simulink model "Source_Dev"  (R2020a)
settings: Solver=ode1  StartTime=0.0  StopTime=3  FixedStep=Time_Step  RelTol=1e-3
values from neighbouring files (symbols this model uses):
  fb = fn    (= 50)    [init.m]
  L0102_L = L0102_X/wb    (= 0.254647908947)    [init.m]
  L0102_R = L0102_R_u*L0102_Zb    (= 8)    [init.m]
  Time_Step = 50e-6    (= 5e-05)    [init.m]
undefined symbols (not defined in the file or in its folder): GRD00_H, GRD00_R, GRD00_TD, GRD00_TN, GRD00_Ub, Source_Lib, Theta0, ThreePhaseVoltageSource, V0, VSC01_id0
libraries: powerlib x54, Control_Lib x6, simulink x5, powerlib_meascontrol x2
(part 1 of 2)
settings Model: Creator=abruyere  LastModifiedBy=abruyere
settings DebuggingCC: UnconnectedInputMsg=none  UnconnectedOutputMsg=none  UnconnectedLineMsg=none
settings SFSimCC: CustomCodeUndefinedFunction=UseInterfaceOnly

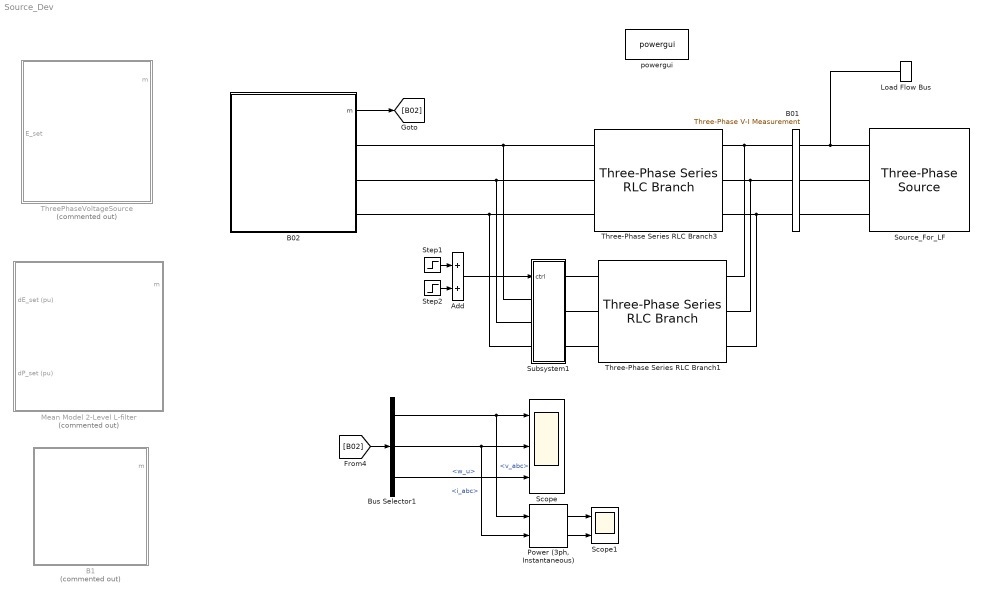
== system Source_Dev ==
  Add : Sum
  B01 : powerlib/Measurements/Three-Phase V-I Measurement  VoltageMeasurement=phase-to-ground  SetLabelV=on  LabelV=B01_v_abc  Vpu=off  VpuLL=off  CurrentMeasurement=yes  SetLabelI=on  LabelI=B01_i_abc  Ipu=off  Pbase=100e6  Vbase=500e3  OutputType=Complex  PhasorSimulation=off  PSBequivalent=0
  B02 : Subsystem  mask(GenericVoltageSource){SourceNature=2 % INERTIAL, fn=50, Sn=10000e3, Un=20000, LFpopup=PQ, P0=350000.4063, Q0=2.0599, U0=10000, V0_pu=1.0045, Theta0_deg=3.9958, H_s=5, R_percent=4, TN=1, TD=2}
      mask prompts: SourceNature "Nature of the source: Choose 1 for infinite source or 2 for inertial source"; fn "Nominal frequency fn [Hz]"; Sn "Nominal apparent power Sn [VA]"; Un "Base nominal voltage Un [V RMS Ph2Ph]"; P0 "Active power P0 [W]"; Q0 "Reactive power Q0 [VAR]"; U0 "Initial voltage U0 [Vrms Ph2Ph]"; V0_pu "Initial pu voltage V0_pu [pu]"; Theta0_deg "Initial angle (°)"; H_s "Inertia H [s]"; R_percent "Droop gain Kp [%]"; TN "Network time constant Lead [s]"; TD "Network time constant Lag [s]"
      mask init:
      | % Update Name of LF bus for internal purpose
      | NameStr = [get_param(gcb,'Name')];% '_LF'];
      | set_param([gcb '/Load Flow Bus'],'ID',NameStr);  
      | 
      | % Base specification
      | fb = fn;                % [Hz] base frequency
      | Sb = Sn;                % [VA] base power
      | Ub = Un;                % [V] base ph2ph voltage
      | Vb = Un/sqrt(3);        % [V] base ph2N voltage
      | Ib = Sb/(3*Vb);         % [A] base current
      | Zb = Vb*Ib;             % [Ohm] base impedance
      | 
      | % Set the frequency droop gain
      | R = R_percent / 100;
      | 
      | % Update mask display:
      | % mo = get_param(gcb,'MaskObject');
      settings: OpenFcn=|
      | set_param(gcb,'MaskType', 'GenericVoltageSource')
      | open_system(gcbh, 'Mask');
      mask TypeOptions SourceNature: 1 % INIFINTE | 2 % INERTIAL
      mask TypeOptions LFpopup: Swing | PQ | PV
      mask Callback LFpopup:
      | % Get the mask parameter values. This is a cell
      | %   array of character vectors.
      | maskStr = get_param(gcb,'LFpopup');
      | p=Simulink.Mask.get(gcb);
      | 
      | % The pop-up menu is the first mask parameter.
      | %   Check the value selected in the pop-up
      | if strcmp(maskStr,'Swing'),
      | 
      |     % Set the visibility of both parameters on when
      |     %   User-defined is selected in the pop-up.
      |     p.getParameter('P0').Visible='off';
      |     p.getParameter('Q0').Visible='off';
      |     p.getParameter('U0').Visible='on';
      |     p.getParameter('Theta0_deg').Visible='on';
      |     set_param([gcb '/Source_For_LF'],'BusType','swing');
      | 
      | elseif strcmp(maskStr,'PQ'),
      | 
      |     % Set the visibility of both parameters on when
      |     %   User-defined is selected in the pop-up.
      |     p.getParameter('P0').Visible='on';
      |     p.getParameter('Q0').Visible='on';
      |     p.getParameter('U0').Visible='off';
      |     p.getParameter('Theta0_deg').Visible='on';
      |     set_param([gcb '/Source_For_LF'],'BusType','PQ');
      | 
      |     % Turn off the visibility of the Value field
      |     %   when User-defined is not selected.
      | else
      | 
      |     % Set the visibility of both parameters on when
      |     %   User-defined is selected in the pop-up.
      |     p.getParameter('P0').Visible='on';
      |     p.getParameter('Q0').Visible='off';
      |     p.getParameter('U0').Visible='on';
      |     p.getParameter('Theta0_deg').Visible='on';
      |     set_param([gcb '/Source_For_LF'],'BusType','PV');
      | 
      | end
      mask DialogControl Container2 Prompt: Nominal specification (for base definition)
      mask DialogControl Container3 Prompt: Loadflow specification
      mask DialogControl Container4_copy Prompt: Inertial source configuration
  B1 : Subsystem  Commented=on  mask(GenericVoltageSource){SourceNature=2 % INERTIAL, fn=50, Sn=1000e3, Un=20e3, P0=199999.317, Q0=4.3832, H_s=5, R_percent=5, V0_pu=0.99767, Theta0_deg=4.0629}
      mask prompts: SourceNature "Nature of the source: Choose 1 for infinite source or 2 for inertial source"; fn "Nominal frequency fn [Hz]"; Sn "Nominal apparent power Sn [VA]"; Un "Base nominal voltage Un [V RMS Ph2Ph]"; P0 "Active power P0 [W]"; Q0 "Reactive power Q0 [VAR]"; H_s "Inertia H [s]"; R_percent "Droop gain Kp [%]"; V0_pu "V0 [pu]"; Theta0_deg "Theta0 [°]"
      mask init:
      | % Update Name of LF bus for internal purpose
      | NameStr = [get_param(gcb,'Name')];% '_LF'];
      | set_param([gcb '/Load Flow Bus'],'ID',NameStr);  
      | 
      | % Base specification
      | fb = fn;                % [Hz] base frequency
      | Sb = Sn;                % [VA] base power
      | Ub = Un;                % [V] base ph2ph voltage
      | Vb = Un/sqrt(3);        % [V] base ph2N voltage
      | Ib = Sb/(3*Vb);         % [A] base current
      | Zb = Vb*Ib;             % [Ohm] base impedance
      | 
      | % Set the frequency droop gain
      | R = R_percent / 100;
      | 
      | % Update mask display:
      | mo = get_param(gcb,'MaskObject');
      | % mo.getDialogControl('LF_V0_str').Prompt = ['V0 = ', num2str(V0),' pu, Angle = ', num2str(V0),'°'];
      settings: OpenFcn=|
      | set_param(gcb,'MaskType', 'GenericVoltageSource')
      | open_system(gcbh, 'Mask');
      mask TypeOptions SourceNature: 1 % INIFINTE | 2 % INERTIAL
      mask DialogControl Container2 Prompt: Nominal specification (for base definition)
      mask DialogControl Container3 Prompt: Setpoint specification (for loadflow)
      mask DialogControl Container4_copy Prompt: Inertial source configuration
      mask DialogControl Container4 Prompt: Info
  Bus Selector1 : BusSelector  OutputSignals=v_abc,i_abc,w_u
  Load Flow Bus : powerlib/Measurements/Load Flow Bus  LConnTagsString=a  Phases=single  Connectors=on one side  ID=B01  Vbase=20e3  Vref=1  Vangle=0  VLF=1  VLFb=1  VLFc=1  angleLF=0  angleLFb=0  angleLFc=0
  Mean Model 2-Level L-filter : Subsystem  Commented=on  AncestorBlock=GFo_Lib/Mean Model 2-Level L-filter  mask(VSC){Parameter33=0, fn=50, Sn=1000e6, Pn=1000e6, Udcn=640e3, Un1=320e3, Un2=400e3, Rt_pu=0.005, Lt_pu=0.15, Lm_pu=500, Rm_pu=500, Tr_PLL=10e-3, Val_Freq_Support=on, R_percent=4, Rv=0.009, W_TVR=60, I_thresh_pu=1, DX_DR=5, Kp_Rvi_pu=0.676, gainpopup=3, wc1=31.4159, mp1=0.0043, wc2=33.3, mp2=0.0033, wc3=2.5, mp3=0.04, T1=0.1210, T2=0.022, LFpopup=PQ, P0=0.5, Q0=0.1, V0=1.0246, Theta0=118.5692}
      mask prompts: Parameter33 "%<MaskType>"; fn "Nominal Frequency (Hz)"; Sn "Nominal Apparent Power (VA)"; Pn "Nominal Power (W)"; Udcn "Nominal DC Voltage (V)"; Un1 "VSC side Nominal Ph-Ph Voltage (V)"; Un2 "Grid side Nominal Ph-Ph Voltage (V)"; Rt_pu "R (pu)"; Lt_pu "L (pu)"; Lm_pu "Rm (pu)"; Rm_pu "Lm (pu)"; Tr_PLL "Time response (s)"; Val_Freq_Support "Frequency Support"; R_percent "Droop Gain (%)"; Rv "Damping Resistance (Rv)"; W_TVR "Dr filter"; I_thresh_pu "Current Threshold (pu)"; Kp_Rvi_pu "Kp_Rvi"; gainpopup "Strategy"; wc1 "wc"; mp1 "mp"; wc2 "wc"; mp2 "mp"; wc3 "wc"; mp3 "mp"; P0 "Initial Active Power (pu)"; Q0 "Initial Reactive Power (pu)"; V0 "Initial Voltage (pu)"; Theta0 "Initial Angle (°)"
      mask init:
      | % Update Name of LF bus for internal purpose
      |     NameStr = [get_param(gcb,'Name')];% '_LF'];
      |     set_param([gcb '/Load Flow Bus'],'ID',NameStr);    
      |     
      | % Base values
      |     fb = fn;
      |     Pb = Pn;
      |     cos_phi_n = Pn/Sn;
      |     Sb = Pb/cos_phi_n;
      |     Vn1 = Un1/sqrt(3);
      |     Vb1 = Vn1;
      |     Vn2 = Un2/sqrt(3);
      |     Vb2 = Vn2;
      |     Ib1 = Sb / 3*Vb1;
      |     Ib2 = Sb / (3*Vb2);
      |     wb = 2*pi*fb;
      |   
      | % PLL derivation of the parameters
      |     wn_PLL=5/Tr_PLL;
      |     zeta_PLL = 1;
      |     Kp_PLL_pu = 2*zeta_PLL*wn_PLL/wb;
      |     Ki_PLL_pu = wn_PLL^2/wb;
      |     
      | % Set the chosen strategy
      |     Chosen_Strategy = gainpopup;
      |     
      | % Set the frequency droop gain
      |     R = R_percent / 100;
      | 
      | % Compute Initial Voltage of VSC 
      | %   from steady-state output transformer model and Loadflow result
      |     
      |     %Initialize correctly the LoadFlow bus parameters connected to PCC
      |     VLF = V0;
      |     ThetaLF = Theta0;
      |     if (LFpopup == 'PQ')
      |         VLF = 1;
      |         ThetaLF = 0;
      |     elseif (LFpopup == 'PV')
      |         VLF = V0;
      |         ThetaLF = 0;        
      |     end
      |     set_param([gcb '/Load Flow Bus'],'Vref',num2str(VLF),'Vangle',num2str(ThetaLF));
      |     
      |     R1_pu = Rt_pu/2;
      |     L1_pu = Lt_pu/2;
      |     R2_pu = Rt_pu/2;
      |     L2_pu = Lt_pu/2;
      |     X1_pu = L1_pu;
      |     X2_pu = L2_pu;
      |     Xm_pu = Lm_pu;
      |     
      |     Zm_pu = 1/(1/Rm_pu+1/(1i*Xm_pu));
      | 
      |     S0=P0+1i*Q0;
      |     I2 = conj(S0)/(V0);
      | 
      |     Vm = (R2_pu+1i*X2_pu)*I2 + V0;
      |     Im = Vm/Zm_pu;
      | 
      |     I1 = I2 + Im;
      |     V1 = (R1_pu+1i*X1_pu) * I1 + Vm;
      | 
      |     Vvsc0 = abs(V1);
      |     Theta_vsc0 = angle(V1) * 180/pi+Theta0;
      |     
      |     Va0 = Vvsc0*sqrt(2)*Vb1*sin(Theta_vsc0*pi/180);
      |     Vb0 = Vvsc0*sqrt(2)*Vb1*sin(Theta_vsc0*pi/180-2*pi/3);
      |     Vc0 = Vvsc0*sqrt(2)*Vb1*sin(Theta_vsc0*pi/180+2*pi/3);
      |     
      | % Generate string to display LF results on Mask
      |     %str_tmp = fprintf("Vvsc0 = %d, Theta_vsc0 = %d°",Vvsc0,Theta_vsc0);
      |     mo = get_param(gcb,'MaskObject');
      |     mo.getDialogControl('LF_vsc_str').Prompt = ['V0 = ', num2str(Vvsc0),' pu, Angle = ', num2str(Theta_vsc0),'°'];
      |     mo.getDialogControl('LF_pcc_str').Prompt = ['V0 = ', num2str(V0),' pu, Angle = ', num2str(Theta0),'°'];
      |     mo.getDialogControl('LF_pcc_Power_str').Prompt = ['P0 = ', num2str(P0),' pu, Q0 = ', num2str(Q0),' pu'];
      |     %set_param([gcb],'LF_str',str_tmp);
      settings: OpenFcn=|
      | NameStr = get_param(gcb,'Name');
      | open_system(gcbh, 'Mask');
      | 
      | h2AllOpenDlgs = DAStudio.ToolRoot.getOpenDialogs;
      | 
      | for i=1:length(h2AllOpenDlgs)
      |     try
      |          %disp(h2AllOpenDlgs(i).getSource.getBlock.Name);
      |         Dialog_block_name = h2AllOpenDlgs(i).getSource.getBlock.Name;
      |          %strcmp(Dialog_block_name, NameStr),
      |         if (strcmp(h2AllOpenDlgs(i).getSource.getBlock.Name, NameStr))
      |             iPos = h2AllOpenDlgs(i).position;
      |             h2AllOpenDlgs(i).position = [iPos(1)   iPos(2)   iPos(3)*1.4   iPos(4)];
      |         end
      |     end
      | end
      mask TypeOptions gainpopup: 1 | 2 | 3
      mask Callback gainpopup:
      | % Get the mask parameter values. This is a cell
      | %   array of character vectors.
      | maskStr = get_param(gcb,'gainpopup');
      | p=Simulink.Mask.get(gcb);
      | 
      | % The pop-up menu is the first mask parameter.
      | %   Check the value selected in the pop-up
      | if strcmp(maskStr,'1'),
      | 
      |     % Set the visibility of both parameters on when
      |     %   User-defined is selected in the pop-up.
      |     p.getDialogControl('Param_Strat_1').Visible='on';
      |     p.getDialogControl('Param_Strat_2').Visible='off';
      |     p.getDialogControl('Param_Strat_3').Visible='off';
      | 
      | elseif strcmp(maskStr,'2'),
      | 
      |     % Set the visibility of both parameters on when
      |     %   User-defined is selected in the pop-up.
      |     p.getDialogControl('Param_Strat_1').Visible='off';
      |     p.getDialogControl('Param_Strat_2').Visible='on';
      |     p.getDialogControl('Param_Strat_3').Visible='off';
      | 
      |     % Turn off the visibility of the Value field
      |     %   when User-defined is not selected.
      | else
      | 
      |     % Set the visibility of both parameters on when
      |     %   User-defined is selected in the pop-up.
      |     p.getDialogControl('Param_Strat_1').Visible='off';
      |     p.getDialogControl('Param_Strat_2').Visible='off';
      |     p.getDialogControl('Param_Strat_3').Visible='on';
      | 
      | end
      mask TypeOptions LFpopup: Swing | PQ | PV
      mask Callback LFpopup:
      | % Get the mask parameter values. This is a cell
      | %   array of character vectors.
      | maskStr = get_param(gcb,'LFpopup');
      | p=Simulink.Mask.get(gcb);
      | 
      | % The pop-up menu is the first mask parameter.
      | %   Check the value selected in the pop-up
      | if strcmp(maskStr,'Swing'),
      | 
      |     % Set the visibility of both parameters on when
      |     %   User-defined is selected in the pop-up.
      |     p.getParameter('P0').Visible='off';
      |     p.getParameter('Q0').Visible='off';
      |     p.getParameter('V0').Visible='on';
      |     p.getParameter('Theta0').Visible='on';
      |     set_param([gcb '/Source_For_LF'],'BusType','swing');
      | 
      | elseif strcmp(maskStr,'PQ'),
      | 
      |     % Set the visibility of both parameters on when
      |     %   User-defined is selected in the pop-up.
      |     p.getParameter('P0').Visible='on';
      |     p.getParameter('Q0').Visible='on';
      |     p.getParameter('V0').Visible='off';
      |     p.getParameter('Theta0').Visible='off';
      |     set_param([gcb '/Source_For_LF'],'BusType','PQ');
      | 
      |     % Turn off the visibility of the Value field
      |     %   when User-defined is not selected.
      | else
      | 
      |     % Set the visibility of both parameters on when
      |     %   User-defined is selected in the pop-up.
      |     p.getParameter('P0').Visible='on';
      |     p.getParameter('Q0').Visible='off';
      |     p.getParameter('V0').Visible='on';
      |     p.getParameter('Theta0').Visible='off';
      |     set_param([gcb '/Source_For_LF'],'BusType','PV');
      | 
      | end
      mask DialogControl Control8 Prompt: (Add text here and link in callback)
      mask DialogControl Nominal_Param Prompt: Nominal Value
      mask DialogControl Container20 Prompt: Output Transformer
      mask DialogControl Control_Param Prompt: Control Parameter
      mask DialogControl Container13 Prompt: PLL
      mask DialogControl Container14 Prompt: Frequency Support
      mask DialogControl Container15 Prompt: Transient Virtual Resistor
      mask DialogControl Container28 Prompt: Virtual Impedance
      mask DialogControl Container18 Prompt: Control Strategy
      mask DialogControl Title_Strat_1 Prompt: Strategy 1
      mask DialogControl Title_Strat_2 Prompt: Strategy 2
      mask DialogControl Title_Strat_3 Prompt: Strategy 3
      mask DialogControl LF_Param Prompt: Loadflow
      mask DialogControl Control4 Prompt: Initial Operating Point
      mask DialogControl Container24 Prompt: VSC side
      mask DialogControl LF_vsc_str Prompt: V0 = 1.0444 pu, Angle = 122.57°
      mask DialogControl Container25 Prompt: PCC
      mask DialogControl LF_pcc_str Prompt: V0 = 1.0246 pu, Angle = 118.5692°
      mask DialogControl LF_pcc_Power_str Prompt: P0 = 0.5 pu, Q0 = 0.1 pu
      mask DialogControl UpdateLoadflow Prompt: Update Loadflow
      mask DialogControl UpdateLoadflow Callback: LoadFlow_VSC
      mask Display:
      | disp('L-Filter');
      | port_label('input',1,'dE_set (pu)');
      | port_label('input',2,'dP_set (pu)');
      | port_label('output',1,'m');
      | port_label('rconn',1,'A');
      | port_label('rconn',2,'B');
      | port_label('rconn',3,'C');
  "Power (3ph, Instantaneous)" : powerlib_meascontrol/Measurements/Power (3ph, Instantaneous)
  Scope : Scope  NumInputPorts=3
  Scope1 : Scope  NumInputPorts=2
  Source_For_LF : powerlib/Electrical Sources/Three-Phase Source  InternalConnection=Yg  VoltagePhases=off  Voltage=(20000)*1  PhaseAngle=0  Voltage_phases=[25e3 25e3 25e3]/sqrt(3)  PhaseAngles_phases=[0 -120 +120]  Frequency=50  NonIdealSource=off  SpecifyImpedance=off  Resistance=0  Inductance=0  ShortCircuitLevel=100e6  BaseVoltage=GRD00_Un  XRratio=7  BusType=swing  Pref=350e3  Qref=0  Prefabc=[10e3, 10e3, 10e3]  Qrefabc=[0, 0, 0]  Qmin=-inf  Qmax=inf
  Step1 : Step  Time=0.5  Before=1  After=0  SampleTime=0
  Step2 : Step  Time=2  SampleTime=0
  Subsystem1 : Subsystem
  Three-Phase Series RLC Branch1 : powerlib/Elements/Three-Phase Series RLC Branch  LConnTagsString=A|B|C  RConnTagsString=A|B|C  BranchType=RL  Resistance=L0102_R*2  Inductance=L0102_L*2  Capacitance=1e-6  Measurements=None
  Three-Phase Series RLC Branch3 : powerlib/Elements/Three-Phase Series RLC Branch  LConnTagsString=A|B|C  RConnTagsString=A|B|C  BranchType=RL  Resistance=L0102_R*2  Inductance=L0102_L*2  Capacitance=1e-6  Measurements=None
  ThreePhaseVoltageSource : Subsystem  Commented=on  AncestorBlock=Source_Lib/ThreePhaseVoltageSource  mask(Inertial_Voltage_source){fb=fb, Sc=1e9, Ub=GRD00_Ub, H_eq=GRD00_H, Droop=GRD00_R, TN=GRD00_TN, TD=GRD00_TD, P0=-0.39869}
      mask prompts: fb "Nominal Frequency (Hz)"; Sc "Nominal Power (VA)"; Ub "Nominal Voltage (V)"; H_eq "Inertial Constant H (s)"; Droop "Droop Gain"; TN "Lead Time Constant"; TD "Lag Time Constant"; P0 "Initial Power"
      mask init:
      | % Update Name of LF bus for internal purpose
      |     NameStr = [get_param(gcb,'Name')];% '_LF'];
      |     set_param([gcb '/Load Flow Bus'],'ID',NameStr);
      | 
      | % Base values
      |     wb=2*pi*fb;
      |     Ib=Sc/(sqrt(3)*Ub);
      |     Vb=Ub/sqrt(3);
      |     e0=Vb;
      |     Theta_e0=0;
      |     P0_VS = P0;
      |   
      | % Parameters
      |     R=Droop;
      mask DialogControl Container5 Prompt: Nominal Values
      mask DialogControl Container16 Prompt: Network Time Constants
  powergui : powerlib/powergui  Priority=1  SimulationMode=Discrete  SampleTime=Time_Step  frequency=65  Iterations=50  frequencyindice=50  Pbase=10000000  ErrMax=1e-4  UnitsV=kV  UnitsW=MW  buscounter=0  FunctionMessages=off  echomessages=off  EnableUseOfTLC=off  CurrentSourceSwitches=off  DisableSnubberDevices=off  DisableRonSwitches=off  DisableVfSwitches=off  DisplayEquations=off  AutomaticDiscreteSolvers=off  SolverType=Tustin/Backward Euler (TBE)  Interpol=off  ExternalGateDelay=off  methode=off  Ts=100  x0status=steady  SPID=on  SwTol=0  HookPort=off  NonlinearTolerance=0  nMaxIteration=15  ContinueOnMaxIteration=off  RestoreLinks=warning  ResistiveCurrentMeasurement=off  Frange=[0:2:500]  Ylog=off  Xlog=on  ShowGrid=off  save=off  variable=ZData  structure=0  ZoomFFT=off  StartTime=0.0  cycles=1  DisplayStyle=1  fundamental=60  FreqAxis=off  MaxFrequency=1000  frequencyindicesteady=1  RmsSteady=1  display=off
  wires:
  Bus Selector1/1 -> "Power (3ph, Instantaneous)"/1, Scope/1  "<v_abc>"
  B02/1(m) -> [B02]
  [B02] -> Bus Selector1/1
  Bus Selector1/2 -> "Power (3ph, Instantaneous)"/2, Scope/2  "<i_abc>"
  Bus Selector1/3 -> Scope/3  "<w_u>"
  "Power (3ph, Instantaneous)"/1 -> Scope1/1
  "Power (3ph, Instantaneous)"/2 -> Scope1/2
  ? -> Mean Model 2-Level L-filter/2(dP_set (pu))
  Add/1 -> Subsystem1/1(ctrl)
  Step1/1 -> Add/1
  Step2/1 -> Add/2
  connections:
  Load Flow Bus/LConn1 -- Source_For_LF/RConn1 -- B01/LConn1
  B01/LConn3 -- Source_For_LF/RConn3
  B01/LConn2 -- Source_For_LF/RConn2
  Three-Phase Series RLC Branch3/LConn1 -- Subsystem1/LConn1 -- B02/RConn1
  Three-Phase Series RLC Branch3/RConn3 -- Three-Phase Series RLC Branch1/RConn3 -- B01/RConn3
  Three-Phase Series RLC Branch3/RConn2 -- Three-Phase Series RLC Branch1/RConn2 -- B01/RConn2
  Three-Phase Series RLC Branch3/LConn2 -- B02/RConn2 -- Subsystem1/LConn2
  Three-Phase Series RLC Branch3/LConn3 -- B02/RConn3 -- Subsystem1/LConn3
  Three-Phase Series RLC Branch3/RConn1 -- Three-Phase Series RLC Branch1/RConn1 -- B01/RConn1
  Subsystem1/RConn3 -- Three-Phase Series RLC Branch1/LConn3
  Subsystem1/RConn2 -- Three-Phase Series RLC Branch1/LConn2
  Subsystem1/RConn1 -- Three-Phase Series RLC Branch1/LConn1

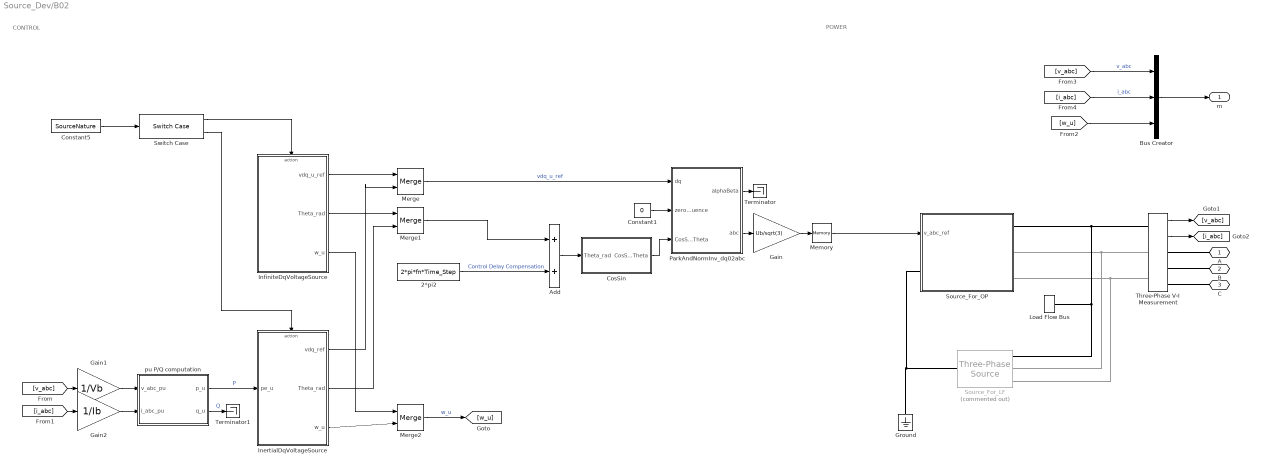
== system Source_Dev/B02 ==
  note: CONTROL
  note: POWER
  " pu P/Q computation" : Subsystem  DialogController=POWERSYS.PowerSysDialog
  2*pi2 : Constant  Value=2*pi*fn*Time_Step
  Add : Sum
  Bus Creator : BusCreator  Inputs=3
  Constant1 : Constant  Value=0
  Constant5 : Constant  Value=SourceNature
  CosSin : Subsystem
  Gain : Gain  Gain=Ub/sqrt(3)
  Gain1 : Gain  Gain=1/Vb
  Gain2 : Gain  Gain=1/Ib
  Ground : powerlib/Elements/Ground  LConnTagsString=a
  InertialDqVoltageSource : Subsystem  TreatAsAtomicUnit=on
  InfiniteDqVoltageSource : Subsystem  TreatAsAtomicUnit=on
  Load Flow Bus : powerlib/Measurements/Load Flow Bus  LConnTagsString=a  Phases=single  Connectors=on one side  ID=B02  Vbase=Un  Vref=1  Vangle=0  VLF=1.005  VLFb=1  VLFc=1  angleLF=3.996  angleLFb=0  angleLFc=0
  Memory : Memory
  Merge : Merge
  Merge1 : Merge
  Merge2 : Merge
  ParkAndNormInv_dq02abc : Subsystem  AncestorBlock=Control_Lib/ParkAndNormInv_dq02abc  TreatAsAtomicUnit=on  mask{referenceAxisMode=Reference axis at 90 degrees behind phase_a, baseUpdateGain=sqrt(3)}
      mask prompts: referenceAxisMode "Chosse reference axis of the angular position"; baseUpdateGain "Gain to update base from dq0 to abc frames"
      mask init:
      | Concordia33 = sqrt(2/3)*[[cos(0) cos(-2*pi/3) cos(-4*pi/3)];
      |                  [-sin(0) -sin(-2*pi/3) -sin(-4*pi/3)];
      |                  [1/sqrt(2) 1/sqrt(2) 1/sqrt(2)];];
      |              
      | Concordia33_inv = transpose(Concordia33);
      mask TypeOptions referenceAxisMode: Reference axis on phase_a | Reference axis at 90 degrees behind phase_a
      mask DialogControl DescGroupVar Prompt: CONFIGURATION
      mask DialogControl Container3 Prompt: Reference axis
      mask DialogControl Container4 Prompt: Base definition
      mask DialogControl Control1 Prompt: Gain = 1.0 : No base update
      mask DialogControl Control1_copy Prompt: Gain = sqrt(3) : 1pu in dq0 frame = 1pu RMS in abc frame
  Source_For_LF : powerlib/Electrical Sources/Three-Phase Source  Commented=on  InternalConnection=Yn  VoltagePhases=off  Voltage=(20000)*1.00454  PhaseAngle=3.9958  Voltage_phases=[25e3 25e3 25e3]/sqrt(3)  PhaseAngles_phases=[0 -120 +120]  Frequency=fb  NonIdealSource=off  SpecifyImpedance=off  Resistance=0  Inductance=0  ShortCircuitLevel=100e6  BaseVoltage=GRD00_Un  XRratio=7  BusType=PQ  Pref=P0  Qref=Q0  Prefabc=[10e3, 10e3, 10e3]  Qrefabc=[0, 0, 0]  Qmin=-inf  Qmax=inf
  Source_For_OP : Subsystem
  Switch Case : SwitchCase  CaseConditions={1, 2}  ShowDefaultCase=off
  Terminator : Terminator
  Terminator1 : Terminator
  Three-Phase V-I Measurement : powerlib/Measurements/Three-Phase V-I Measurement  VoltageMeasurement=phase-to-ground  SetLabelV=off  LabelV=v_abc  Vpu=off  VpuLL=off  CurrentMeasurement=yes  SetLabelI=off  LabelI=i_abc  Ipu=off  Pbase=100e6  Vbase=500e3  OutputType=Complex  PhasorSimulation=off  PSBequivalent=0
  A : PMIOPort  Side=Right
  B : PMIOPort  Port=2  Side=Right
  C : PMIOPort  Port=3  Side=Right
  m : Outport  VectorParamsAs1DForOutWhenUnconnected=off
  wires:
  ParkAndNormInv_dq02abc/2(abc) -> Gain/1
  Constant1/1 -> ParkAndNormInv_dq02abc/2(zeroSequence)
  ParkAndNormInv_dq02abc/1(alphaBeta) -> Terminator/1
  Gain/1 -> Memory/1
  Constant5/1 -> Switch Case/1
  Switch Case/1 -> InfiniteDqVoltageSource/Action
  InfiniteDqVoltageSource/1(vdq_u_ref) -> Merge/1
  InertialDqVoltageSource/1(vdq_ref) -> Merge/2
  Merge/1 -> ParkAndNormInv_dq02abc/1(dq)  "vdq_u_ref"
  InfiniteDqVoltageSource/2(Theta_rad) -> Merge1/1
  InertialDqVoltageSource/2(Theta_rad) -> Merge1/2
  Switch Case/2 -> InertialDqVoltageSource/Action
  [v_abc] -> Gain1/1
  [i_abc] -> Gain2/1
  Gain1/1 -> " pu P/Q computation"/1(v_abc_pu)
  Gain2/1 -> " pu P/Q computation"/2(i_abc_pu)
  CosSin/1(CosSinTheta) -> ParkAndNormInv_dq02abc/3(CosSinTheta)
  " pu P/Q computation"/2(q_u) -> Terminator1/1  "Q"
  " pu P/Q computation"/1(p_u) -> InertialDqVoltageSource/1(pe_u)  "P"
  Memory/1 -> Source_For_OP/1(v_abc_ref)
  Add/1 -> CosSin/1(Theta_rad)
  Merge1/1 -> Add/1
  2*pi2/1 -> Add/2  "Control Delay Compensation"
  InertialDqVoltageSource/3(w_u) -> Merge2/2
  [v_abc] -> Bus Creator/1  "v_abc"
  [i_abc] -> Bus Creator/2  "i_abc"
  [w_u] -> Bus Creator/3
  InfiniteDqVoltageSource/3(w_u) -> Merge2/1
  Merge2/1 -> [w_u]  "w_u"
  Bus Creator/1 -> m/1
  Three-Phase V-I Measurement/1 -> [v_abc]
  Three-Phase V-I Measurement/2 -> [i_abc]
  connections:
  Source_For_LF/RConn2 -- Three-Phase V-I Measurement/LConn2 -- Source_For_OP/RConn2
  Source_For_OP/LConn1 -- Ground/LConn1 -- Source_For_LF/LConn1
  Source_For_LF/RConn3 -- Three-Phase V-I Measurement/LConn3 -- Source_For_OP/RConn3
  Source_For_OP/RConn1 -- Source_For_LF/RConn1 -- Load Flow Bus/LConn1 -- Three-Phase V-I Measurement/LConn1
  Three-Phase V-I Measurement/RConn1 -- A/RConn1
  Three-Phase V-I Measurement/RConn2 -- B/RConn1
  Three-Phase V-I Measurement/RConn3 -- C/RConn1

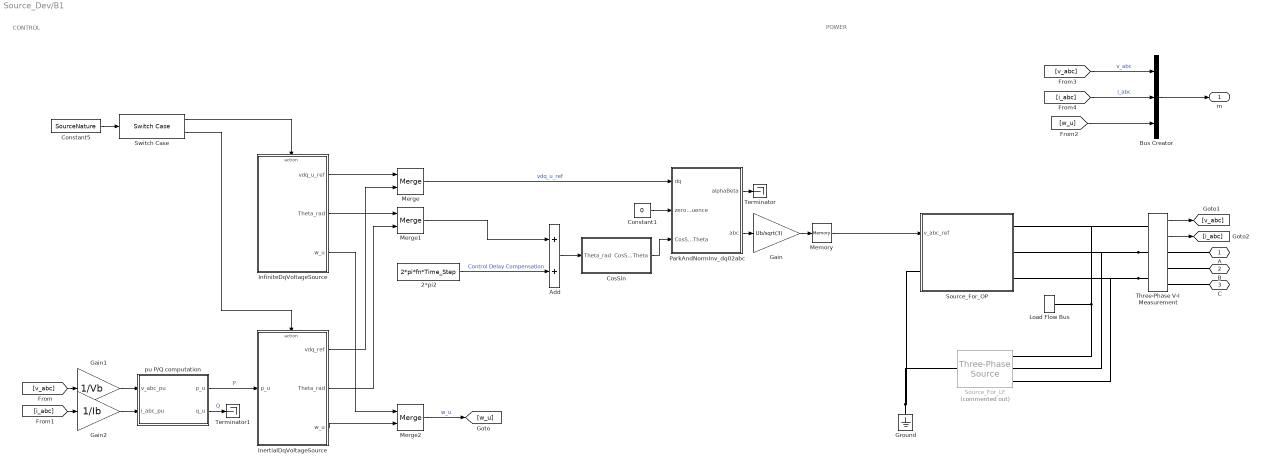
== system Source_Dev/B1 ==
  note: POWER
  note: CONTROL
  " pu P/Q computation" : Subsystem  DialogController=POWERSYS.PowerSysDialog
  2*pi2 : Constant  Value=2*pi*fn*Time_Step
  Add : Sum
  Bus Creator : BusCreator  Inputs=3
  Constant1 : Constant  Value=0
  Constant5 : Constant  Value=SourceNature
  CosSin : Subsystem
  Gain : Gain  Gain=Ub/sqrt(3)
  Gain1 : Gain  Gain=1/Vb
  Gain2 : Gain  Gain=1/Ib
  Ground : powerlib/Elements/Ground  LConnTagsString=a
  InertialDqVoltageSource : Subsystem  TreatAsAtomicUnit=on
  InfiniteDqVoltageSource : Subsystem  TreatAsAtomicUnit=on
  Load Flow Bus : powerlib/Measurements/Load Flow Bus  LConnTagsString=a  Phases=single  Connectors=on one side  ID=B1  Vbase=Un  Vref=1  Vangle=0  VLF=0.9977  VLFb=1  VLFc=1  angleLF=4.063  angleLFb=0  angleLFc=0
  Memory : Memory
  Merge : Merge
  Merge1 : Merge
  Merge2 : Merge
  ParkAndNormInv_dq02abc : Subsystem  AncestorBlock=Control_Lib/ParkAndNormInv_dq02abc  TreatAsAtomicUnit=on  mask{referenceAxisMode=Reference axis at 90 degrees behind phase_a, baseUpdateGain=sqrt(3)}
      mask prompts: referenceAxisMode "Chosse reference axis of the angular position"; baseUpdateGain "Gain to update base from dq0 to abc frames"
      mask init: same as Source_Dev/B02/ParkAndNormInv_dq02abc
      mask TypeOptions referenceAxisMode: Reference axis on phase_a | Reference axis at 90 degrees behind phase_a
      mask DialogControl DescGroupVar Prompt: CONFIGURATION
      mask DialogControl Container3 Prompt: Reference axis
      mask DialogControl Container4 Prompt: Base definition
      mask DialogControl Control1 Prompt: Gain = 1.0 : No base update
      mask DialogControl Control1_copy Prompt: Gain = sqrt(3) : 1pu in dq0 frame = 1pu RMS in abc frame
  Source_For_LF : powerlib/Electrical Sources/Three-Phase Source  Commented=on  InternalConnection=Yn  VoltagePhases=off  Voltage=(20000)*0.997669  PhaseAngle=4.0629  Voltage_phases=[25e3 25e3 25e3]/sqrt(3)  PhaseAngles_phases=[0 -120 +120]  Frequency=fb  NonIdealSource=off  SpecifyImpedance=off  Resistance=0  Inductance=0  ShortCircuitLevel=100e6  BaseVoltage=GRD00_Un  XRratio=7  BusType=PQ  Pref=P0  Qref=Q0  Prefabc=[10e3, 10e3, 10e3]  Qrefabc=[0, 0, 0]  Qmin=-inf  Qmax=inf
  Source_For_OP : Subsystem
  Switch Case : SwitchCase  CaseConditions={1, 2}  ShowDefaultCase=off
  Terminator : Terminator
  Terminator1 : Terminator
  Three-Phase V-I Measurement : powerlib/Measurements/Three-Phase V-I Measurement  VoltageMeasurement=phase-to-ground  SetLabelV=off  LabelV=v_abc  Vpu=off  VpuLL=off  CurrentMeasurement=yes  SetLabelI=off  LabelI=i_abc  Ipu=off  Pbase=100e6  Vbase=500e3  OutputType=Complex  PhasorSimulation=off  PSBequivalent=0
  A : PMIOPort  Side=Right
  B : PMIOPort  Port=2  Side=Right
  C : PMIOPort  Port=3  Side=Right
  m : Outport  VectorParamsAs1DForOutWhenUnconnected=off
  wires:
  Three-Phase V-I Measurement/2 -> [i_abc]
  Three-Phase V-I Measurement/1 -> [v_abc]
  Bus Creator/1 -> m/1
  Merge2/1 -> [w_u]  "w_u"
  InfiniteDqVoltageSource/3(w_u) -> Merge2/1
  [w_u] -> Bus Creator/3
  [i_abc] -> Bus Creator/2  "i_abc"
  [v_abc] -> Bus Creator/1  "v_abc"
  InertialDqVoltageSource/3(w_u) -> Merge2/2
  2*pi2/1 -> Add/2  "Control Delay Compensation"
  Merge1/1 -> Add/1
  Add/1 -> CosSin/1(Theta_rad)
  Memory/1 -> Source_For_OP/1(v_abc_ref)
  " pu P/Q computation"/1(p_u) -> InertialDqVoltageSource/1(p_u)  "P"
  " pu P/Q computation"/2(q_u) -> Terminator1/1  "Q"
  CosSin/1(CosSinTheta) -> ParkAndNormInv_dq02abc/3(CosSinTheta)
  Gain2/1 -> " pu P/Q computation"/2(i_abc_pu)
  Gain1/1 -> " pu P/Q computation"/1(v_abc_pu)
  [i_abc] -> Gain2/1
  [v_abc] -> Gain1/1
  Switch Case/2 -> InertialDqVoltageSource/Action
  InertialDqVoltageSource/2(Theta_rad) -> Merge1/2
  InfiniteDqVoltageSource/2(Theta_rad) -> Merge1/1
  Merge/1 -> ParkAndNormInv_dq02abc/1(dq)  "vdq_u_ref"
  InertialDqVoltageSource/1(vdq_ref) -> Merge/2
  InfiniteDqVoltageSource/1(vdq_u_ref) -> Merge/1
  Switch Case/1 -> InfiniteDqVoltageSource/Action
  Constant5/1 -> Switch Case/1
  Gain/1 -> Memory/1
  ParkAndNormInv_dq02abc/1(alphaBeta) -> Terminator/1
  Constant1/1 -> ParkAndNormInv_dq02abc/2(zeroSequence)
  ParkAndNormInv_dq02abc/2(abc) -> Gain/1
  connections:
  Three-Phase V-I Measurement/RConn3 -- C/RConn1
  Three-Phase V-I Measurement/RConn2 -- B/RConn1
  Three-Phase V-I Measurement/RConn1 -- A/RConn1
  Three-Phase V-I Measurement/LConn1 -- Source_For_OP/RConn1 -- Load Flow Bus/LConn1 -- Source_For_LF/RConn1
  Three-Phase V-I Measurement/LConn3 -- Source_For_OP/RConn3 -- Source_For_LF/RConn3
  Ground/LConn1 -- Source_For_OP/LConn1 -- Source_For_LF/LConn1
  Three-Phase V-I Measurement/LConn2 -- Source_For_OP/RConn2 -- Source_For_LF/RConn2

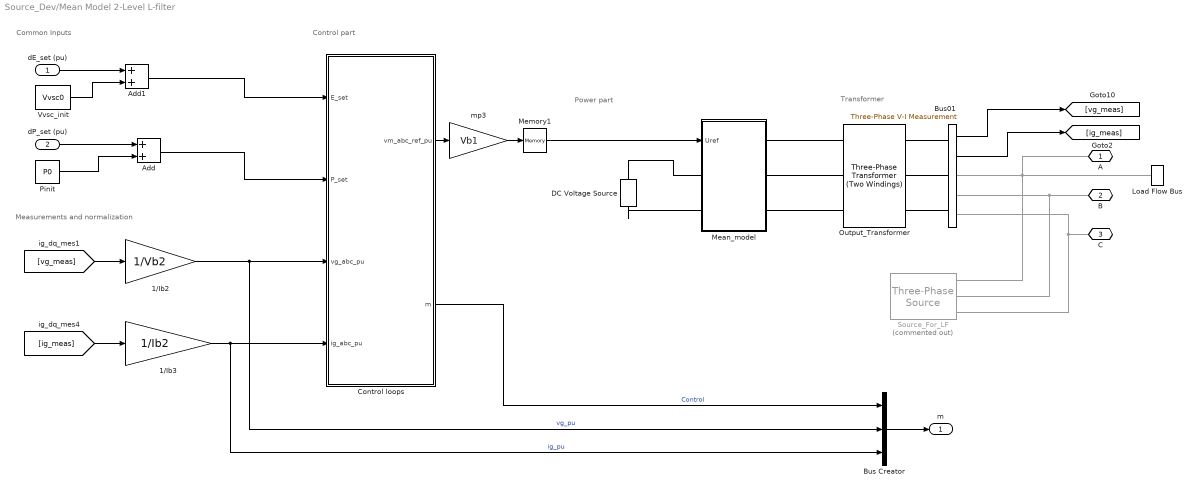
== system Source_Dev/Mean Model 2-Level L-filter ==
  note: Transformer
  note: Common Inputs
  note: Power part
  note: Measurements and normalization
  note: Control part
  dE_set (pu) : Inport
  dP_set (pu) : Inport  Port=2
  1/Ib2 : Gain  Gain=1/Vb2
  1/Ib3 : Gain  Gain=1/Ib2
  Add : Sum
  Add1 : Sum
  Bus Creator : BusCreator  Inputs=3
  Bus01 : powerlib/Measurements/Three-Phase V-I Measurement  VoltageMeasurement=phase-to-ground  SetLabelV=off  LabelV=Vabc  Vpu=off  VpuLL=off  CurrentMeasurement=yes  SetLabelI=off  LabelI=Iabc  Ipu=off  Pbase=100e6  Vbase=500e3  OutputType=Complex  PhasorSimulation=off  PSBequivalent=0
  Control loops : Subsystem
  DC Voltage Source : powerlib/Electrical Sources/DC Voltage Source  Amplitude=Udcn  Measurements=Voltage
  Load Flow Bus : powerlib/Measurements/Load Flow Bus  LConnTagsString=a  Phases=single  Connectors=on one side  ID=Mean Model 2-Level L-filter  Vbase=Un2  Vref=1.0246  Vangle=118.5692  VLF=1.001  VLFb=1  VLFc=1  angleLF=0.5724  angleLFb=0  angleLFc=0
  Mean_model : Subsystem
  Memory1 : Memory  InitialCondition=[Va0 Vb0 Vc0]
  Output_Transformer : powerlib/Elements/Three-Phase Transformer (Two Windings)  Winding1Connection=Yg  Winding2Connection=Yg  CoreType=Three single-phase transformers  SetSaturation=off  Hysteresis=off  DataFile='hysteresis'  SetInitialFlux=off  Measurements=None  UNITS=pu  NominalPower=[Sn , fb]  Winding1=[Un1 , Rt_pu/2 , Lt_pu/2]  Winding2=[Un2 , Rt_pu/2 , Lt_pu/2]  Rm=Rm_pu  Lm=Lm_pu  L0=0.5  Saturation=[ 0,0 ; 0.0024,1.2 ; 1.0,1.52 ]  InitialFluxes=[ 0.8 , -0.8 , 0.7 ]  BreakLoop=off  DiscreteSolver=Trapezoidal iterative  DataType=off  TransfoNumber=1
  Pinit : Constant  Value=P0
  Source_For_LF : powerlib/Electrical Sources/Three-Phase Source  Commented=on  InternalConnection=Yg  VoltagePhases=off  Voltage=Un2  PhaseAngle=90  Voltage_phases=[25e3 25e3 25e3]/sqrt(3)  PhaseAngles_phases=[0 -120 +120]  Frequency=fb  NonIdealSource=off  SpecifyImpedance=off  Resistance=0  Inductance=0  ShortCircuitLevel=100e6  BaseVoltage=Un  XRratio=7  BusType=swing  Pref=P0*Sb  Qref=Q0*Sb  Prefabc=[10e3, 10e3, 10e3]  Qrefabc=[0, 0, 0]  Qmin=-inf  Qmax=inf
  Vvsc_init : Constant  Value=Vvsc0
  mp3 : Gain  Gain=Vb1
  A : PMIOPort  Side=Right
  B : PMIOPort  Port=2  Side=Right
  C : PMIOPort  Port=3  Side=Right
  m : Outport  VectorParamsAs1DForOutWhenUnconnected=off
  wires:
  Add/1 -> Control loops/2(P_set)
  Control loops/2(m) -> Bus Creator/1  "Control"
  mp3/1 -> Memory1/1
  1/Ib3/1 -> Bus Creator/3, Control loops/4(ig_abc_pu)  "ig_pu"
  1/Ib2/1 -> Bus Creator/2, Control loops/3(vg_abc_pu)  "vg_pu"
  Bus Creator/1 -> m/1
  [vg_meas] -> 1/Ib2/1
  Control loops/1(vm_abc_ref_pu) -> mp3/1
  Add1/1 -> Control loops/1(E_set)
  Memory1/1 -> Mean_model/1(Uref)
  dP_set (pu)/1 -> Add/1
  Pinit/1 -> Add/2
  Vvsc_init/1 -> Add1/2
  Bus01/1 -> [vg_meas]
  dE_set (pu)/1 -> Add1/1
  Bus01/2 -> [ig_meas]
  [ig_meas] -> 1/Ib3/1
  connections:
  DC Voltage Source/LConn1 -- Mean_model/LConn2
  Output_Transformer/RConn1 -- Bus01/LConn1
  Output_Transformer/RConn2 -- Bus01/LConn2
  DC Voltage Source/RConn1 -- Mean_model/LConn1
  Output_Transformer/RConn3 -- Bus01/LConn3
  Source_For_LF/RConn2 -- B/RConn1 -- Bus01/RConn2
  Mean_model/RConn1 -- Output_Transformer/LConn1
  Mean_model/RConn2 -- Output_Transformer/LConn2
  Mean_model/RConn3 -- Output_Transformer/LConn3
  Source_For_LF/RConn1 -- Load Flow Bus/LConn1 -- A/RConn1 -- Bus01/RConn1
  Source_For_LF/RConn3 -- C/RConn1 -- Bus01/RConn3

== system Source_Dev/Subsystem1 ==
  ctrl : Inport
  Breaker1 : powerlib/Elements/Breaker  InitialState=1  SwitchingTimes="[1/60  5/60]"  External=on  BreakerResistance=0.001  SnubberResistance=1e6  SnubberCapacitance=inf  Measurements=None  MoreParameters=on  NoBreakLoop=off
  Breaker2 : powerlib/Elements/Breaker  InitialState=1  SwitchingTimes="[1/60  5/60]"  External=on  BreakerResistance=0.001  SnubberResistance=1e6  SnubberCapacitance=inf  Measurements=None  MoreParameters=on  NoBreakLoop=off
  Breaker3 : powerlib/Elements/Breaker  InitialState=1  SwitchingTimes="[1/60  5/60]"  External=on  BreakerResistance=0.001  SnubberResistance=1e6  SnubberCapacitance=inf  Measurements=None  MoreParameters=on  NoBreakLoop=off
  a : PMIOPort  Side=Left
  b : PMIOPort  Port=2  Side=Left
  c : PMIOPort  Port=3  Side=Left
  A : PMIOPort  Port=4  Side=Right
  B : PMIOPort  Port=5  Side=Right
  C : PMIOPort  Port=6  Side=Right
  wires:
  ctrl/1 -> Breaker3/1, Breaker1/1, Breaker2/1
  connections:
  Breaker3/RConn1 -- C/RConn1
  Breaker2/LConn1 -- a/RConn1
  Breaker3/LConn1 -- c/RConn1
  Breaker2/RConn1 -- A/RConn1
  Breaker1/LConn1 -- b/RConn1
  Breaker1/RConn1 -- B/RConn1

== system Source_Dev/ThreePhaseVoltageSource ==
  E_set : Inport
  Bus00 : powerlib/Measurements/Three-Phase V-I Measurement  VoltageMeasurement=phase-to-ground  SetLabelV=off  LabelV=Vabc  Vpu=off  VpuLL=off  CurrentMeasurement=yes  SetLabelI=off  LabelI=Iabc  Ipu=off  Pbase=100e6  Vbase=500e3  OutputType=Complex  PhasorSimulation=off  PSBequivalent=0
  Load Flow Bus : powerlib/Measurements/Load Flow Bus  LConnTagsString=a  Phases=single  Connectors=on one side  ID=ThreePhaseVoltageSource  Vbase=Ub  Vref=1  Vangle=0  VLF=1  VLFb=1  VLFc=1  angleLF=0  angleLFb=0  angleLFc=0
  Mean_model : Subsystem
  Simplified SG : Subsystem
  Source_For_LF : powerlib/Electrical Sources/Three-Phase Source  Commented=on  InternalConnection=Yg  VoltagePhases=off  Voltage=(400000)*1  PhaseAngle=0  Voltage_phases=[25e3 25e3 25e3]/sqrt(3)  PhaseAngles_phases=[0 -120 +120]  Frequency=fb  NonIdealSource=on  SpecifyImpedance=off  Resistance=0  Inductance=0  ShortCircuitLevel=100e6  BaseVoltage=GRD00_Un  XRratio=7  BusType=swing  Pref=P0  Qref=Q0  Prefabc=[10e3, 10e3, 10e3]  Qrefabc=[0, 0, 0]  Qmin=-inf  Qmax=inf
  A : PMIOPort  Side=Right
  B : PMIOPort  Port=2  Side=Right
  C : PMIOPort  Port=3  Side=Right
  "m " : Outport  VectorParamsAs1DForOutWhenUnconnected=off
  wires:
  Bus00/2 -> [GRD00_i_abc]
  Bus00/1 -> [GRD00_U_abc]
  Simplified SG/2(m) -> "m "/1
  [GRD00_i_abc] -> Simplified SG/2(ig_mes)
  Simplified SG/1(vg_abc) -> Mean_model/1(u_abc)
  E_set/1 -> Simplified SG/3(E_set)
  [GRD00_U_abc] -> Simplified SG/1(eg_mes)
  connections:
  C/RConn1 -- Bus00/RConn3
  B/RConn1 -- Bus00/RConn2
  A/RConn1 -- Bus00/RConn1
  Mean_model/RConn1 -- Bus00/LConn1 -- Load Flow Bus/LConn1 -- Source_For_LF/RConn1
  Mean_model/RConn2 -- Bus00/LConn2 -- Source_For_LF/RConn2
  Mean_model/RConn3 -- Bus00/LConn3 -- Source_For_LF/RConn3

== system Source_Dev/B02/ pu P//Q computation ==
  v_abc_pu : Inport  PortDimensions=3
  i_abc_pu : Inport  Port=2  PortDimensions=3
  Demux : Demux  Outputs=3
      settings: DisplayOption=none
  Mux : Mux  Inputs=3
  Product1 : Product  InputSameDT=on  SaturateOnIntegerOverflow=on  OutDataTypeStr=Inherit: Same as first input
  Product3 : Product  InputSameDT=on  SaturateOnIntegerOverflow=on  OutDataTypeStr=Inherit: Same as first input
  Sum : Sum  Inputs=+-  InputSameDT=on  SaturateOnIntegerOverflow=on  OutDataTypeStr=Inherit: Same as first input
  Sum1 : Sum  Inputs=1  InputSameDT=on  SaturateOnIntegerOverflow=on  OutDataTypeStr=Inherit: Same as first input
  Sum4 : Sum  Inputs=1  InputSameDT=on  SaturateOnIntegerOverflow=on  OutDataTypeStr=Inherit: Same as first input
  Sum5 : Sum  Inputs=+-  InputSameDT=on  SaturateOnIntegerOverflow=on  OutDataTypeStr=Inherit: Same as first input
  Sum6 : Sum  Inputs=+-  InputSameDT=on  SaturateOnIntegerOverflow=on  OutDataTypeStr=Inherit: Same as first input
  pu->V : Gain  Gain=1/sqrt(3)  SaturateOnIntegerOverflow=on  OutDataTypeStr=Inherit: Same as input  ParamDataTypeStr=Inherit: Same as input
  pu->V1 : Gain  Gain=1/3  SaturateOnIntegerOverflow=on  OutDataTypeStr=Inherit: Same as input  ParamDataTypeStr=Inherit: Same as input
  pu->V2 : Gain  Gain=1/3  SaturateOnIntegerOverflow=on  OutDataTypeStr=Inherit: Same as input  ParamDataTypeStr=Inherit: Same as input
  p_u : Outport  VectorParamsAs1DForOutWhenUnconnected=off
  q_u : Outport  Port=2  VectorParamsAs1DForOutWhenUnconnected=off
  wires:
  pu->V2/1 -> q_u/1
  pu->V1/1 -> p_u/1
  Sum1/1 -> pu->V/1
  Product3/1 -> Sum1/1
  Product1/1 -> Sum4/1
  v_abc_pu/1 -> Product1/1, Demux/1
  i_abc_pu/1 -> Product1/2, Product3/2
  Sum4/1 -> pu->V1/1
  Demux/1 -> Sum/1, Sum6/2
  Demux/2 -> Sum/2, Sum5/1
  Demux/3 -> Sum5/2, Sum6/1
  Sum/1 -> Mux/3
  Sum5/1 -> Mux/1
  Sum6/1 -> Mux/2
  Mux/1 -> Product3/1
  pu->V/1 -> pu->V2/1  "Q"

== system Source_Dev/B02/CosSin ==
  Theta_rad : Inport
  Mux : Mux  Inputs=2
  Trigonometric Function : Trigonometry
  Trigonometric Function1 : Trigonometry  Operator=cos
  CosSinTheta : Outport  VectorParamsAs1DForOutWhenUnconnected=off
  wires:
  Theta_rad/1 -> Trigonometric Function/1, Trigonometric Function1/1
  Trigonometric Function/1 -> Mux/2
  Mux/1 -> CosSinTheta/1
  Trigonometric Function1/1 -> Mux/1

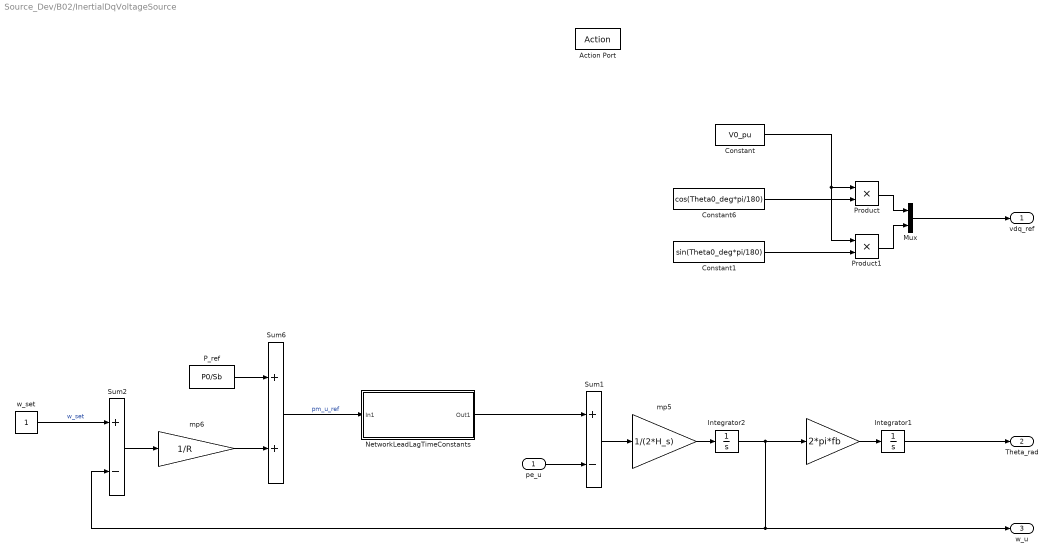
== system Source_Dev/B02/InertialDqVoltageSource ==
  pe_u : Inport
  Action Port : ActionPort  ActionPortLabel=case [ 2 ]:
  " " : Gain  Gain=2*pi*fb
  Constant : Constant  Value=V0_pu
  Constant1 : Constant  Value=sin(Theta0_deg*pi/180)
  Constant6 : Constant  Value=cos(Theta0_deg*pi/180)
  Integrator1 : Integrator
  Integrator2 : Integrator  InitialCondition=1
  Mux : Mux  Inputs=2
  NetworkLeadLagTimeConstants : Subsystem
  P_ref : Constant  Value=P0/Sb
  Product : Product
  Product1 : Product
  Sum1 : Sum  Inputs=+-
  Sum2 : Sum  Inputs=+-
  Sum6 : Sum
  mp5 : Gain  Gain=1/(2*H_s)
  mp6 : Gain  Gain=1/R
  w_set : Constant
  vdq_ref : Outport  VectorParamsAs1DForOutWhenUnconnected=off
  Theta_rad : Outport  Port=2  VectorParamsAs1DForOutWhenUnconnected=off
  w_u : Outport  Port=3  VectorParamsAs1DForOutWhenUnconnected=off
  wires:
  mp5/1 -> Integrator2/1
  mp6/1 -> Sum6/2
  Sum6/1 -> NetworkLeadLagTimeConstants/1(In1)  "pm_u_ref"
  Integrator2/1 -> Sum2/2, w_u/1, " "/1
  P_ref/1 -> Sum6/1
  Sum2/1 -> mp6/1
  Sum1/1 -> mp5/1
  " "/1 -> Integrator1/1
  pe_u/1 -> Sum1/2
  w_set/1 -> Sum2/1  "w_set"
  Integrator1/1 -> Theta_rad/1
  Constant1/1 -> Product1/2
  Constant6/1 -> Product/2
  Constant/1 -> Product1/1, Product/1
  Product1/1 -> Mux/2
  Product/1 -> Mux/1
  Mux/1 -> vdq_ref/1
  NetworkLeadLagTimeConstants/1(Out1) -> Sum1/1

== system Source_Dev/B02/InfiniteDqVoltageSource ==
  Action Port : ActionPort  ActionPortLabel=case [ 1 ]:
  Constant : Constant  Value=V0_pu
  Constant1 : Constant  Value=sin(Theta0_deg*pi/180)
  Constant4 : Constant
  Constant6 : Constant  Value=cos(Theta0_deg*pi/180)
  Gain : Gain  Gain=2*pi*fn
  Integrator : Integrator
  Mux : Mux  Inputs=2
  Product : Product
  Product1 : Product
  vdq_u_ref : Outport  VectorParamsAs1DForOutWhenUnconnected=off
  Theta_rad : Outport  Port=2  VectorParamsAs1DForOutWhenUnconnected=off
  w_u : Outport  Port=3  VectorParamsAs1DForOutWhenUnconnected=off
  wires:
  Constant1/1 -> Product1/2
  Gain/1 -> Integrator/1
  Product/1 -> Mux/1
  Constant6/1 -> Product/2
  Constant/1 -> Product1/1, Product/1
  Product1/1 -> Mux/2
  Integrator/1 -> Theta_rad/1
  Mux/1 -> vdq_u_ref/1
  Constant4/1 -> w_u/1, Gain/1

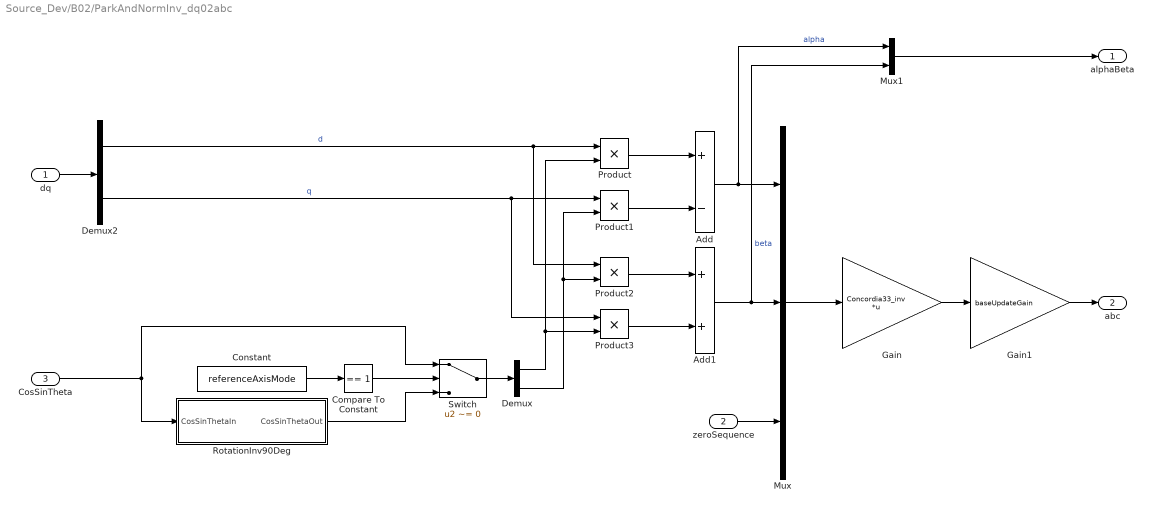
== system Source_Dev/B02/ParkAndNormInv_dq02abc ==
  dq : Inport
  zeroSequence : Inport  Port=2
  CosSinTheta : Inport  Port=3
  Add : Sum  Inputs=+-
  Add1 : Sum
  Compare To Constant : simulink/Logic and Bit Operations/Compare To Constant  relop===  const=1  OutDataTypeStr=boolean
  Constant : Constant  Value=referenceAxisMode  OutDataTypeStr=uint16
  Demux : Demux  Outputs=2
  Demux2 : Demux  Outputs=2
  Gain : Gain  Gain=Concordia33_inv  Multiplication=Matrix(K*u)
  Gain1 : Gain  Gain=baseUpdateGain
  Mux : Mux  Inputs=3
  Mux1 : Mux  Inputs=2
  Product{,1..3} (4 alike) : Product
  RotationInv90Deg : Subsystem  VariantControl=ROTATIONINV90DEG
  Switch : Switch  Criteria=u2 ~= 0
  alphaBeta : Outport  VectorParamsAs1DForOutWhenUnconnected=off
  abc : Outport  Port=2  VectorParamsAs1DForOutWhenUnconnected=off
  wires:
  Gain1/1 -> abc/1
  Constant/1 -> Compare To Constant/1
  RotationInv90Deg/1(CosSinThetaOut) -> Switch/3
  Demux/1 -> Product3/2, Product/2
  Mux/1 -> Gain/1
  Switch/1 -> Demux/1
  Demux/2 -> Product2/2, Product1/2
  Mux1/1 -> alphaBeta/1
  Product/1 -> Add/1
  Demux2/2 -> Product1/1, Product3/1  "q"
  Add1/1 -> Mux/2, Mux1/2  "beta"
  Product1/1 -> Add/2
  Compare To Constant/1 -> Switch/2
  Product2/1 -> Add1/1
  Product3/1 -> Add1/2
  CosSinTheta/1 -> Switch/1, RotationInv90Deg/1(CosSinThetaIn)
  dq/1 -> Demux2/1
  zeroSequence/1 -> Mux/3
  Demux2/1 -> Product/1, Product2/1  "d"
  Add/1 -> Mux/1, Mux1/1  "alpha"
  Gain/1 -> Gain1/1

== system Source_Dev/B02/Source_For_OP ==
  v_abc_ref : Inport
  Controlled Voltage Source1 : powerlib/Electrical Sources/Controlled Voltage Source  Initialize=off  Source_Type=AC  Amplitude=V0*Ub*sqrt(2/3)*sin(Theta0)  Phase=(Theta0*180/pi)  Frequency=fb  Measurements=None
  Controlled Voltage Source2 : powerlib/Electrical Sources/Controlled Voltage Source  Initialize=off  Source_Type=AC  Amplitude=V0*Ub*sqrt(2/3)*sin(Theta0-2*pi/3)  Phase=(Theta0*180/pi)-120  Frequency=fb  Measurements=None
  Controlled Voltage Source3 : powerlib/Electrical Sources/Controlled Voltage Source  Initialize=off  Source_Type=AC  Amplitude=V0*Ub*sqrt(2/3)*sin(Theta0-4*pi/3)  Phase=(Theta0*180/pi)+120  Frequency=fb  Measurements=None
  Demux : Demux  Outputs=3
  Step : Step  Time=1e-9  SampleTime=0
  Subsystem3 : Subsystem
  Three-Phase Source1 : powerlib/Electrical Sources/Three-Phase Source  InternalConnection=Yn  VoltagePhases=off  Voltage=V0_pu*Ub  PhaseAngle=Theta0_deg  Voltage_phases=[25e3 25e3 25e3]/sqrt(3)  PhaseAngles_phases=[0 -120 +120]  Frequency=fb  NonIdealSource=off  SpecifyImpedance=off  Resistance=0.8929  Inductance=16.58e-3  ShortCircuitLevel=100e6  BaseVoltage=25e3  XRratio=7  BusType=swing  Pref=10e3  Qref=0  Prefabc=[10e3, 10e3, 10e3]  Qrefabc=[0, 0, 0]  Qmin=-inf  Qmax=inf
  A : PMIOPort  Side=Right
  B : PMIOPort  Port=2  Side=Right
  C : PMIOPort  Port=3  Side=Right
  N : PMIOPort  Port=4  Side=Left
  wires:
  Demux/2 -> Controlled Voltage Source2/1
  v_abc_ref/1 -> Demux/1
  Demux/1 -> Controlled Voltage Source1/1
  Demux/3 -> Controlled Voltage Source3/1
  Step/1 -> Subsystem3/1(switch)
  connections:
  Controlled Voltage Source3/LConn1 -- Three-Phase Source1/LConn1 -- N/RConn1 -- Controlled Voltage Source2/LConn1 -- Controlled Voltage Source1/LConn1
  Subsystem3/RConn1 -- A/RConn1
  Subsystem3/RConn2 -- B/RConn1
  Subsystem3/RConn3 -- C/RConn1
  Controlled Voltage Source1/RConn1 -- Subsystem3/LConn1
  Controlled Voltage Source2/RConn1 -- Subsystem3/LConn2
  Controlled Voltage Source3/RConn1 -- Subsystem3/LConn3
  Three-Phase Source1/RConn1 -- Subsystem3/LConn4
  Three-Phase Source1/RConn2 -- Subsystem3/LConn5
  Three-Phase Source1/RConn3 -- Subsystem3/LConn6

== system Source_Dev/B1/ pu P//Q computation ==
  v_abc_pu : Inport  PortDimensions=3
  i_abc_pu : Inport  Port=2  PortDimensions=3
  Demux : Demux  Outputs=3
      settings: DisplayOption=none
  Mux : Mux  Inputs=3
  Product1 : Product  InputSameDT=on  SaturateOnIntegerOverflow=on  OutDataTypeStr=Inherit: Same as first input
  Product3 : Product  InputSameDT=on  SaturateOnIntegerOverflow=on  OutDataTypeStr=Inherit: Same as first input
  Sum : Sum  Inputs=+-  InputSameDT=on  SaturateOnIntegerOverflow=on  OutDataTypeStr=Inherit: Same as first input
  Sum1 : Sum  Inputs=1  InputSameDT=on  SaturateOnIntegerOverflow=on  OutDataTypeStr=Inherit: Same as first input
  Sum4 : Sum  Inputs=1  InputSameDT=on  SaturateOnIntegerOverflow=on  OutDataTypeStr=Inherit: Same as first input
  Sum5 : Sum  Inputs=+-  InputSameDT=on  SaturateOnIntegerOverflow=on  OutDataTypeStr=Inherit: Same as first input
  Sum6 : Sum  Inputs=+-  InputSameDT=on  SaturateOnIntegerOverflow=on  OutDataTypeStr=Inherit: Same as first input
  pu->V : Gain  Gain=1/sqrt(3)  SaturateOnIntegerOverflow=on  OutDataTypeStr=Inherit: Same as input  ParamDataTypeStr=Inherit: Same as input
  pu->V1 : Gain  Gain=1/3  SaturateOnIntegerOverflow=on  OutDataTypeStr=Inherit: Same as input  ParamDataTypeStr=Inherit: Same as input
  pu->V2 : Gain  Gain=1/3  SaturateOnIntegerOverflow=on  OutDataTypeStr=Inherit: Same as input  ParamDataTypeStr=Inherit: Same as input
  p_u : Outport  VectorParamsAs1DForOutWhenUnconnected=off
  q_u : Outport  Port=2  VectorParamsAs1DForOutWhenUnconnected=off
  wires:
  pu->V/1 -> pu->V2/1  "Q"
  Mux/1 -> Product3/1
  Sum6/1 -> Mux/2
  Sum5/1 -> Mux/1
  Sum/1 -> Mux/3
  Demux/3 -> Sum6/1, Sum5/2
  Demux/2 -> Sum5/1, Sum/2
  Demux/1 -> Sum6/2, Sum/1
  Sum4/1 -> pu->V1/1
  i_abc_pu/1 -> Product3/2, Product1/2
  v_abc_pu/1 -> Demux/1, Product1/1
  Product1/1 -> Sum4/1
  Product3/1 -> Sum1/1
  Sum1/1 -> pu->V/1
  pu->V1/1 -> p_u/1
  pu->V2/1 -> q_u/1

== system Source_Dev/B1/CosSin ==
  Theta_rad : Inport
  Mux : Mux  Inputs=2
  Trigonometric Function : Trigonometry
  Trigonometric Function1 : Trigonometry  Operator=cos
  CosSinTheta : Outport  VectorParamsAs1DForOutWhenUnconnected=off
  wires:
  Trigonometric Function1/1 -> Mux/1
  Mux/1 -> CosSinTheta/1
  Trigonometric Function/1 -> Mux/2
  Theta_rad/1 -> Trigonometric Function1/1, Trigonometric Function/1

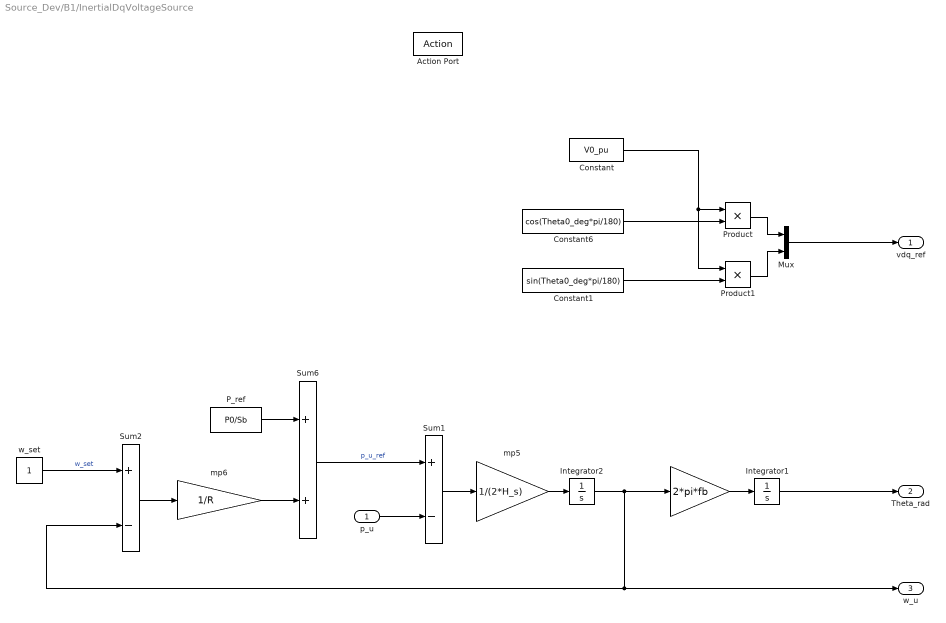
== system Source_Dev/B1/InertialDqVoltageSource ==
  p_u : Inport
  Action Port : ActionPort  ActionPortLabel=case [ 2 ]:
  " " : Gain  Gain=2*pi*fb
  Constant : Constant  Value=V0_pu
  Constant1 : Constant  Value=sin(Theta0_deg*pi/180)
  Constant6 : Constant  Value=cos(Theta0_deg*pi/180)
  Integrator1 : Integrator
  Integrator2 : Integrator  InitialCondition=1
  Mux : Mux  Inputs=2
  P_ref : Constant  Value=P0/Sb
  Product : Product
  Product1 : Product
  Sum1 : Sum  Inputs=+-
  Sum2 : Sum  Inputs=+-
  Sum6 : Sum
  mp5 : Gain  Gain=1/(2*H_s)
  mp6 : Gain  Gain=1/R
  w_set : Constant
  vdq_ref : Outport  VectorParamsAs1DForOutWhenUnconnected=off
  Theta_rad : Outport  Port=2  VectorParamsAs1DForOutWhenUnconnected=off
  w_u : Outport  Port=3  VectorParamsAs1DForOutWhenUnconnected=off
  wires:
  Mux/1 -> vdq_ref/1
  Product/1 -> Mux/1
  Product1/1 -> Mux/2
  Constant/1 -> Product/1, Product1/1
  Constant6/1 -> Product/2
  Constant1/1 -> Product1/2
  Integrator1/1 -> Theta_rad/1
  w_set/1 -> Sum2/1  "w_set"
  p_u/1 -> Sum1/2
  " "/1 -> Integrator1/1
  Sum1/1 -> mp5/1
  Sum2/1 -> mp6/1
  P_ref/1 -> Sum6/1
  Integrator2/1 -> " "/1, w_u/1, Sum2/2
  Sum6/1 -> Sum1/1  "p_u_ref"
  mp6/1 -> Sum6/2
  mp5/1 -> Integrator2/1

== system Source_Dev/B1/InfiniteDqVoltageSource ==
  Action Port : ActionPort  ActionPortLabel=case [ 1 ]:
  Constant : Constant  Value=V0_pu
  Constant1 : Constant  Value=sin(Theta0_deg*pi/180)
  Constant4 : Constant
  Constant6 : Constant  Value=cos(Theta0_deg*pi/180)
  Gain : Gain  Gain=2*pi*fn
  Integrator : Integrator
  Mux : Mux  Inputs=2
  Product : Product
  Product1 : Product
  vdq_u_ref : Outport  VectorParamsAs1DForOutWhenUnconnected=off
  Theta_rad : Outport  Port=2  VectorParamsAs1DForOutWhenUnconnected=off
  w_u : Outport  Port=3  VectorParamsAs1DForOutWhenUnconnected=off
  wires:
  Constant4/1 -> Gain/1, w_u/1
  Mux/1 -> vdq_u_ref/1
  Integrator/1 -> Theta_rad/1
  Product1/1 -> Mux/2
  Constant/1 -> Product/1, Product1/1
  Constant6/1 -> Product/2
  Product/1 -> Mux/1
  Gain/1 -> Integrator/1
  Constant1/1 -> Product1/2
